simulink model "NDI_and_CA_Model"  (R2012b)
settings: Solver=FixedStepDiscrete  StartTime=0.0  StopTime=inf  FixedStep=T_sim  MaxStep=0.01  RelTol=1e-5
values from neighbouring files (symbols this model uses):
  A_x = 0.015    [SetupComplete.m]
  A_y = A_x    (= 0.015)    [SetupComplete.m]
  A_z = 0.16    [SetupComplete.m]
  C_x = 1.2    [SetupComplete.m]
  C_y = C_x    (= 1.2)    [SetupComplete.m]
  C_z = 2.2    [SetupComplete.m]
  CG_0 = [0,0,0.02]'    [SetupComplete.m]
  eta_23 = deg2rad(-1.42)    [Run3Copter.m]
  g = 9.81    [SetupComplete.m]
  h_M = 0.064    [SetupComplete.m]
  I_BAC_0 = [ Ix,0,Ixz;0,Iy,0;Ixz,0,Iz]    [SetupComplete.m]
  l = 0.345    [SetupComplete.m]
  l_arm = 0.264    [SetupComplete.m]
  m = 3.51    [SetupComplete.m]
  m_0 = 2.61    [SetupComplete.m]
  m_M = 0.300    (= 0.3)    [SetupComplete.m]
  rho = 1.15    [SetupComplete.m]
  Rotation_sign = [ 1,-1,-1]    [SetupComplete.m]
  throtle_1 = 0.512    [Run3Copter.m]
  throtle_23 = throtle_1/cos(eta_23)    [Run3Copter.m]
  Throttle_Hover = X(1)/16    [SetupComplete.m]
libraries: XXCopter_C x24, simulink_extras x21, aerolibutil x3
(part 2 of 2)

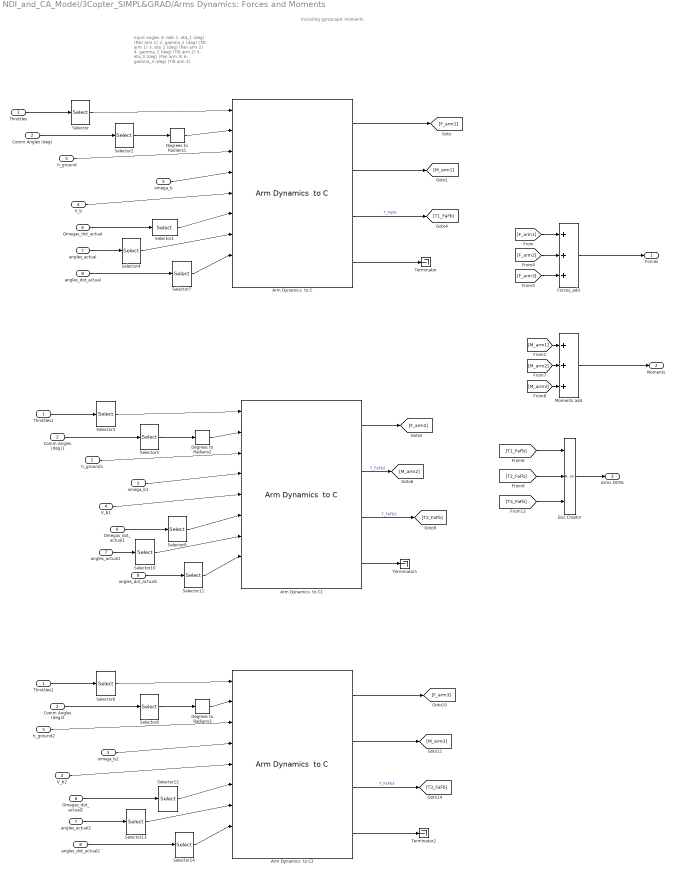
== system NDI_and_CA_Model/3Copter_SIMPL&GRAD/Arms Dynamics: Forces and Moments ==
  note: Including gyroscopic moments
  note: Input angles in rads
      |
      | 1. eta_1 (deg)  (Pan arm 1)
      | 2. gamma_1 (deg)  (Tilt arm 1)
      |
      | 3. eta_2 (deg)  (Pan arm 2)
      | 4. gamma_2 (deg)  (Tilt arm 2)
      |
      | 5. eta_3 (deg)  (Pan arm  3)
      | 6. gamma_3 (deg)  (Tilt arm 3)
  Throttles : Inport
  Comm Angles (deg) : Inport  Port=2
  omega_b : Inport  Port=3
  V_b : Inport  Port=4
  h_ground : Inport  Port=5
  Omegas_dot_actual : Inport  Port=6
  angles_actual : Inport  Port=7
  angles_dot_actual : Inport  Port=8
  Arm Dynamics  to C : XXCopter_C/Arm Dynamics  to C  Rot_sign=Rotation_sign(1)  arm_hub_pos=l*[1;0;0]  Arm_axis=[l_arm;0;0]  arm_num=1  eta_dir=[1;0;0]  gamma_dir=[0;1;0]  J_T=J_T  J_FA=J_FA  h=h  switch_val=direct_feedforward  omega_n=35  xi=1.45  eta_inf_lim=deg2rad(-180)  eta_sup_lim=deg2rad(180)  gamma_inf_lim=deg2rad(-90)  gamma_sup_lim=deg2rad(30)
      link override ESC+Motor Dynamcis  to C/2-D Torque-Throttle-Omega Map: BreakpointsForDimension1=Torque_TTO_vec  BreakpointsForDimension2=Throtle_TTO_vec
  Arm Dynamics  to C1 : XXCopter_C/Arm Dynamics  to C  Rot_sign=Rotation_sign(2)  arm_hub_pos=l*[-1/2;sqrt(3)/2;0]  Arm_axis=[0;l_arm;0]  arm_num=2  eta_dir=[0;1;0]  gamma_dir=[1;0;0]  J_T=J_T  J_FA=J_FA  h=h  switch_val=direct_feedforward  omega_n=35  xi=1.45  eta_inf_lim=deg2rad(-180)  eta_sup_lim=deg2rad(180)  gamma_inf_lim=deg2rad(-30)  gamma_sup_lim=deg2rad(90)
  Arm Dynamics  to C2 : XXCopter_C/Arm Dynamics  to C  Rot_sign=Rotation_sign(3)  arm_hub_pos=l*[-1/2;-sqrt(3)/2;0]  Arm_axis=[0;-l_arm;0]  arm_num=3  eta_dir=[0;1;0]  gamma_dir=[1;0;0]  J_T=J_T  J_FA=J_FA  h=h  switch_val=direct_feedforward  omega_n=35  xi=1.45  eta_inf_lim=deg2rad(-180)  eta_sup_lim=deg2rad(180)  gamma_inf_lim=deg2rad(-90)  gamma_sup_lim=deg2rad(30)
  Bus Creator : BusCreator  Inputs=3
  Comm Angles (deg)1 : InportShadow  Port=2
  Comm Angles (deg)2 : InportShadow  Port=2
  Degrees to Radians1 : simulink_extras/Transformations/Degrees to Radians
  Degrees to Radians2 : simulink_extras/Transformations/Degrees to Radians
  Degrees to Radians3 : simulink_extras/Transformations/Degrees to Radians
  Forces_add : Sum  Inputs=+++
  Moments add : Sum  Inputs=+++
  Omegas_dot_actual1 : InportShadow  Port=6
  Omegas_dot_actual2 : InportShadow  Port=6
  Selector : Selector  IndexMode=Zero-based  InputPortWidth=3  Indices=0
  Selector1 : Selector  IndexMode=Zero-based  InputPortWidth=3  Indices=0
  Selector10 : Selector  IndexMode=Zero-based  InputPortWidth=6  Indices=[2,3]
  Selector11 : Selector  IndexMode=Zero-based  InputPortWidth=6  Indices=[2,3]
  Selector12 : Selector  IndexMode=Zero-based  InputPortWidth=3  Indices=2
  Selector13 : Selector  IndexMode=Zero-based  InputPortWidth=6  Indices=[4,5]
  Selector14 : Selector  IndexMode=Zero-based  InputPortWidth=6  Indices=[4,5]
  Selector2 : Selector  IndexMode=Zero-based  InputPortWidth=6  Indices=[0,1]
  Selector3 : Selector  IndexMode=Zero-based  InputPortWidth=3
  Selector4 : Selector  IndexMode=Zero-based  InputPortWidth=6  Indices=[0,1]
  Selector5 : Selector  IndexMode=Zero-based  InputPortWidth=6  Indices=[2,3]
  Selector6 : Selector  IndexMode=Zero-based  InputPortWidth=3  Indices=2
  Selector7 : Selector  IndexMode=Zero-based  InputPortWidth=6  Indices=[0,1]
  Selector8 : Selector  IndexMode=Zero-based  InputPortWidth=6  Indices=[4,5]
  Selector9 : Selector  IndexMode=Zero-based  InputPortWidth=3
  Terminator : Terminator
  Terminator1 : Terminator
  Terminator2 : Terminator
  Throttles1 : InportShadow
  Throttles2 : InportShadow
  V_b1 : InportShadow  Port=4
  V_b2 : InportShadow  Port=4
  angles_actual1 : InportShadow  Port=7
  angles_actual2 : InportShadow  Port=7
  angles_dot_actual1 : InportShadow  Port=8
  angles_dot_actual2 : InportShadow  Port=8
  h_ground1 : InportShadow  Port=5
  h_ground2 : InportShadow  Port=5
  omega_b1 : InportShadow  Port=3
  omega_b2 : InportShadow  Port=3
  Forces : Outport
  Moments : Outport  Port=2
  Arms DCMs : Outport  Port=3
  wires:
  Throttles/1 -> Selector/1
  Selector/1 -> Arm Dynamics  to C/1
  V_b/1 -> Arm Dynamics  to C/5
  Forces_add/1 -> Forces/1
  Moments add/1 -> Moments/1
  h_ground/1 -> Arm Dynamics  to C/3
  Arm Dynamics  to C/1 -> [F_arm1]
  Arm Dynamics  to C/2 -> [M_arm1]
  [F_arm1] -> Forces_add/1
  [M_arm1] -> Moments add/1
  omega_b/1 -> Arm Dynamics  to C/4
  [F_arm2] -> Forces_add/2
  [F_arm3] -> Forces_add/3
  [M_arm3] -> Moments add/3
  [M_arm2] -> Moments add/2
  Degrees to Radians1/1 -> Arm Dynamics  to C/2
  Comm Angles (deg)/1 -> Selector2/1
  Selector2/1 -> Degrees to Radians1/1
  Arm Dynamics  to C/3 -> [T1_FaFb]  "T_FaFb"
  Throttles1/1 -> Selector3/1
  Selector3/1 -> Arm Dynamics  to C1/1
  V_b1/1 -> Arm Dynamics  to C1/5
  h_ground1/1 -> Arm Dynamics  to C1/3
  omega_b1/1 -> Arm Dynamics  to C1/4
  Degrees to Radians2/1 -> Arm Dynamics  to C1/2
  Comm Angles (deg)1/1 -> Selector5/1
  Selector5/1 -> Degrees to Radians2/1
  Arm Dynamics  to C1/3 -> [T2_FaFb]  "T_FaFb2"
  Throttles2/1 -> Selector6/1
  Selector6/1 -> Arm Dynamics  to C2/1
  V_b2/1 -> Arm Dynamics  to C2/5
  h_ground2/1 -> Arm Dynamics  to C2/3
  Arm Dynamics  to C2/1 -> [F_arm3]
  Arm Dynamics  to C2/2 -> [M_arm3]
  omega_b2/1 -> Arm Dynamics  to C2/4
  Degrees to Radians3/1 -> Arm Dynamics  to C2/2
  Comm Angles (deg)2/1 -> Selector8/1
  Selector8/1 -> Degrees to Radians3/1
  Arm Dynamics  to C2/3 -> [T3_FaFb]  "T_FaFb3"
  Arm Dynamics  to C/4 -> Terminator/1
  Arm Dynamics  to C1/4 -> Terminator1/1
  Arm Dynamics  to C2/4 -> Terminator2/1
  Arm Dynamics  to C1/1 -> [F_arm2]
  Arm Dynamics  to C1/2 -> [M_arm2]  "T_FaFb2"
  Bus Creator/1 -> Arms DCMs/1
  [T1_FaFb] -> Bus Creator/1
  [T2_FaFb] -> Bus Creator/2
  [T3_FaFb] -> Bus Creator/3
  Omegas_dot_actual/1 -> Selector1/1
  Selector1/1 -> Arm Dynamics  to C/6
  angles_actual/1 -> Selector4/1
  Selector4/1 -> Arm Dynamics  to C/7
  angles_dot_actual/1 -> Selector7/1
  Selector7/1 -> Arm Dynamics  to C/8
  Omegas_dot_actual1/1 -> Selector9/1
  Selector9/1 -> Arm Dynamics  to C1/6
  Selector10/1 -> Arm Dynamics  to C1/7
  angles_dot_actual1/1 -> Selector11/1
  angles_actual1/1 -> Selector10/1
  Selector11/1 -> Arm Dynamics  to C1/8
  Omegas_dot_actual2/1 -> Selector12/1
  Selector12/1 -> Arm Dynamics  to C2/6
  Selector13/1 -> Arm Dynamics  to C2/7
  angles_dot_actual2/1 -> Selector14/1
  angles_actual2/1 -> Selector13/1
  Selector14/1 -> Arm Dynamics  to C2/8

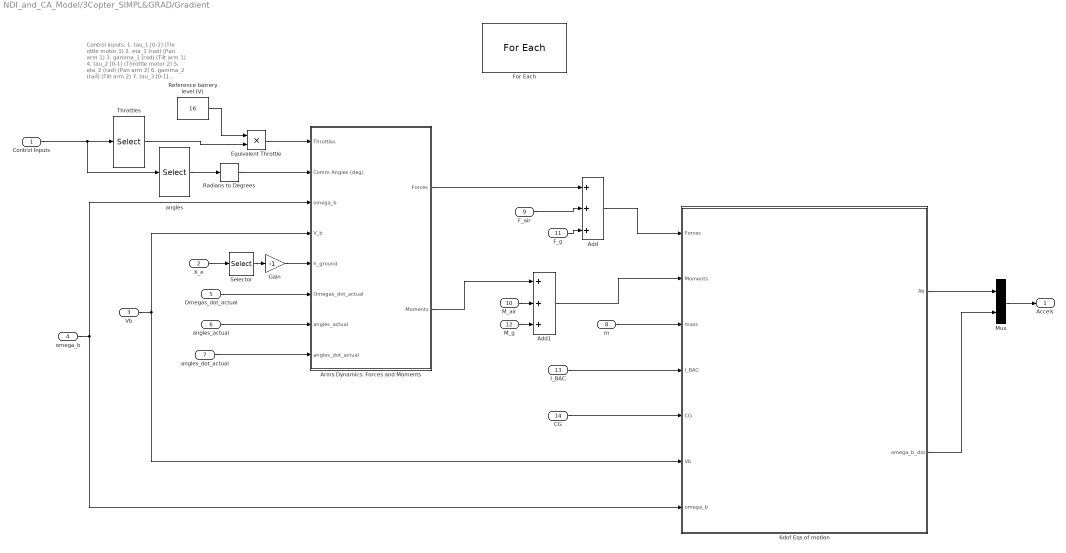
== system NDI_and_CA_Model/3Copter_SIMPL&GRAD/Gradient ==
  note: Control inputs:
      | 1. tau_1 [0-1] (Thr ottle motor 1)
      | 2. eta_1 (rad)  (Pan arm 1)
      | 3. gamma_1 (rad)  (Tilt arm 1)
      |
      | 4. tau_2 [0-1] (Throttle motor 2)
      | 5. eta_2 (rad)  (Pan arm 2)
      | 6. gamma_2 (rad)  (Tilt arm 2)
      |
      | 7. tau_3 [0-1] (Throttle motor 3)
      | 8. eta_3 (rad)  (Pan arm  3)
      | 9. gamma_3 (rad)  (Tilt arm 3)
  "Control Inputs " : Inport  Partition=on  PartitionDimension=1  PartitionWidth=9
  X_e : Inport  Port=2  Partition=off
  Vb : Inport  Port=3  Partition=off
  omega_b : Inport  Port=4  Partition=off
  Omegas_dot_actual : Inport  Port=5  Partition=off
  angles_actual : Inport  Port=6  Partition=off
  angles_dot_actual : Inport  Port=7  Partition=off
  " m" : Inport  Port=8  Partition=off
  F_air : Inport  Port=9  Partition=off
  M_air : Inport  Port=10  Partition=off
  F_g : Inport  Port=11  Partition=off
  M_g : Inport  Port=12  Partition=off
  I_BAC : Inport  Port=13  Partition=off
  CG : Inport  Port=14  Partition=off
  6dof Eqs of motion : Subsystem  TreatAsAtomicUnit=on
  Add : Sum  Inputs=+++
  Add1 : Sum  Inputs=+++
  Arms Dynamics: Forces and Moments : Subsystem  TreatAsAtomicUnit=on
  Equivalent Throttle : Product  Inputs=**
  For Each : ForEach  DisableCoverage=on  IndexMode=One-based
  Gain : Gain  Gain=-1
  Mux : Mux  Inputs=[3,3]
  Radians to Degrees : simulink_extras/Transformations/Radians to Degrees
  Reference batrery level (V) : Constant  Value=16
  Selector : Selector  IndexMode=Zero-based  InputPortWidth=3  Indices=2
  Throttles : Selector  IndexMode=Zero-based  InputPortWidth=9  Indices=[0,3,6]
  "angles " : Selector  IndexMode=Zero-based  InputPortWidth=9  Indices=[1,2,4,5,7,8]
  Accels : Outport  ConcatenationDimension=2
  wires:
  " m"/1 -> 6dof Eqs of motion/3(mass)
  Vb/1 -> 6dof Eqs of motion/6(Vb), Arms Dynamics: Forces and Moments/4(V_b)
  omega_b/1 -> Arms Dynamics: Forces and Moments/3(omega_b), 6dof Eqs of motion/7(omega_b)
  X_e/1 -> Selector/1
  Selector/1 -> Gain/1
  Gain/1 -> Arms Dynamics: Forces and Moments/5(h_ground)
  F_air/1 -> Add/2
  Arms Dynamics: Forces and Moments/1(Forces) -> Add/1
  F_g/1 -> Add/3
  Arms Dynamics: Forces and Moments/2(Moments) -> Add1/1
  M_g/1 -> Add1/3
  M_air/1 -> Add1/2
  Throttles/1 -> Equivalent Throttle/2
  "Control Inputs "/1 -> Throttles/1, "angles "/1
  "angles "/1 -> Radians to Degrees/1
  Add/1 -> 6dof Eqs of motion/1(Forces)
  CG/1 -> 6dof Eqs of motion/5(CG)
  I_BAC/1 -> 6dof Eqs of motion/4(I_BAC)
  Equivalent Throttle/1 -> Arms Dynamics: Forces and Moments/1(Throttles)
  Reference batrery level (V)/1 -> Equivalent Throttle/1
  Add1/1 -> 6dof Eqs of motion/2(Moments)
  6dof Eqs of motion/2(omega_b_dot) -> Mux/2
  Omegas_dot_actual/1 -> Arms Dynamics: Forces and Moments/6(Omegas_dot_actual)
  angles_dot_actual/1 -> Arms Dynamics: Forces and Moments/8(angles_dot_actual)
  angles_actual/1 -> Arms Dynamics: Forces and Moments/7(angles_actual)
  6dof Eqs of motion/1(Ab) -> Mux/1
  Mux/1 -> Accels/1
  Radians to Degrees/1 -> Arms Dynamics: Forces and Moments/2(Comm Angles (deg))

== system NDI_and_CA_Model/3Copter_SIMPL&GRAD/Mass Properties ==
  Arms DCMs : Inport
  CG_0 : Inport  Port=2
  m_0 : Inport  Port=3
  m : Inport  Port=4
  m_M : Inport  Port=5
  I_BAC_0 : Inport  Port=6
  Arm Inertia : MATLAB Function  TreatAsAtomicUnit=on
      settings: PermitHierarchicalResolution=ParametersOnly
  Bus Selector : BusSelector  OutputSignals=T_FaFb,T_FaFb2,T_FaFb3
  CG position : Sum
  Divide : Product  Inputs=*/
  Divide1 : Product  Inputs=**
  Divide2 : Product  Inputs=/*
  Divide3 : Product  Inputs=**
  Motors Pos sum : Sum  Inputs=+++
  Total I_BAC : Sum
  I_BAC : Outport
  CG : Outport  Port=2
  wires:
  Arms DCMs/1 -> Bus Selector/1
  Bus Selector/3 -> Arm Inertia/3(T3_FAFb)  "<T_FaFb3>"
  Bus Selector/2 -> Arm Inertia/2(T2_FAFb)  "<T_FaFb2>"
  Bus Selector/1 -> Arm Inertia/1(T1_FAFb)  "<T_FaFb>"
  Total I_BAC/1 -> I_BAC/1
  m_0/1 -> Divide/1
  m/1 -> Divide/2, Divide2/1
  CG_0/1 -> Divide1/1
  Divide/1 -> Divide1/2
  m_M/1 -> Divide2/2
  CG position/1 -> CG/1
  Divide1/1 -> CG position/1
  Motors Pos sum/1 -> Divide3/1
  Divide2/1 -> Divide3/2
  Divide3/1 -> CG position/2
  Arm Inertia/3(r2_M) -> Motors Pos sum/2
  Arm Inertia/4(r3_M) -> Motors Pos sum/1
  Arm Inertia/1(I_M) -> Total I_BAC/2
  I_BAC_0/1 -> Total I_BAC/1
  Arm Inertia/2(r1_M) -> Motors Pos sum/3

== system NDI_and_CA_Model/3Copter_SIMPL&GRAD/Normalize Quaternion ==
  q : Inport
  Demux : Demux
  Math Function : Math  Operator=reciprocal  SaturateOnIntegerOverflow=on
  Mux : Mux
  Product{,1..3} (4 alike) : Product  Inputs=**
  Quaternion Modulus : aerolibutil/Quaternion Modulus
  normal(q) : Outport
  wires:
  Product3/1 -> Mux/4
  Product2/1 -> Mux/3
  Product1/1 -> Mux/2
  Product/1 -> Mux/1
  Quaternion Modulus/1 -> Math Function/1
  q/1 -> Demux/1, Quaternion Modulus/1
  Mux/1 -> normal(q)/1
  Demux/1 -> Product/1
  Demux/2 -> Product1/1
  Demux/3 -> Product2/1
  Demux/4 -> Product3/1
  Math Function/1 -> Product3/2, Product2/2, Product/2, Product1/2

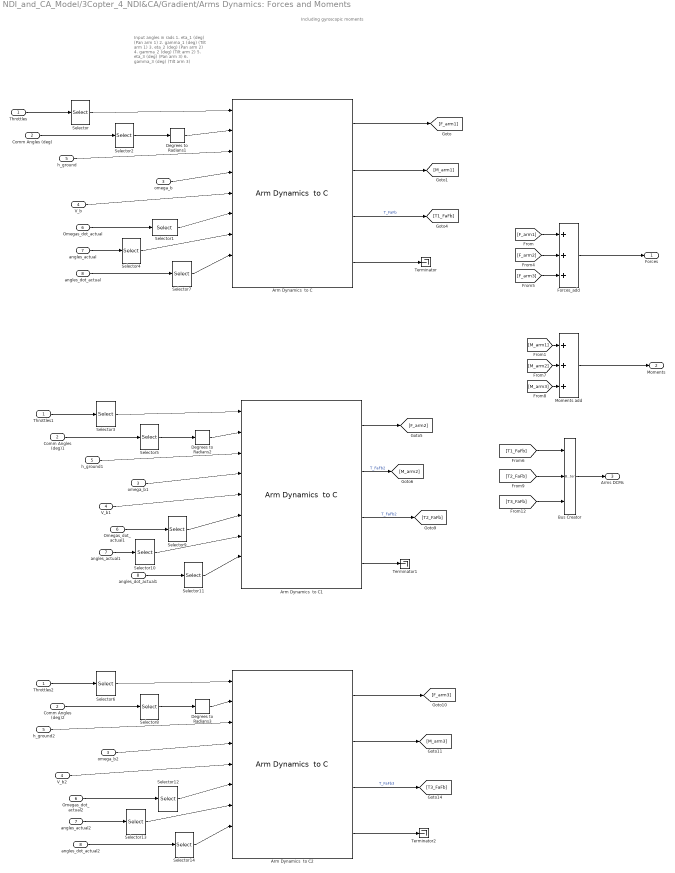
== system NDI_and_CA_Model/3Copter_4_NDI&CA/Gradient/Arms Dynamics: Forces and Moments ==
  note: Including gyroscopic moments
  note: Input angles in rads
      |
      | 1. eta_1 (deg)  (Pan arm 1)
      | 2. gamma_1 (deg)  (Tilt arm 1)
      |
      | 3. eta_2 (deg)  (Pan arm 2)
      | 4. gamma_2 (deg)  (Tilt arm 2)
      |
      | 5. eta_3 (deg)  (Pan arm  3)
      | 6. gamma_3 (deg)  (Tilt arm 3)
  Throttles : Inport
  Comm Angles (deg) : Inport  Port=2
  omega_b : Inport  Port=3
  V_b : Inport  Port=4
  h_ground : Inport  Port=5
  Omegas_dot_actual : Inport  Port=6
  angles_actual : Inport  Port=7
  angles_dot_actual : Inport  Port=8
  Arm Dynamics  to C : XXCopter_C/Arm Dynamics  to C  Rot_sign=Rotation_sign(1)  arm_hub_pos=l*[1;0;0]  Arm_axis=[l_arm;0;0]  arm_num=1  eta_dir=[1;0;0]  gamma_dir=[0;1;0]  J_T=J_T  J_FA=J_FA  h=h  switch_val=direct_feedforward  omega_n=35  xi=1.45  eta_inf_lim=deg2rad(-180)  eta_sup_lim=deg2rad(180)  gamma_inf_lim=deg2rad(-90)  gamma_sup_lim=deg2rad(30)
      link override ESC+Motor Dynamcis  to C/2-D Torque-Throttle-Omega Map: BreakpointsForDimension1=Torque_TTO_vec  BreakpointsForDimension2=Throtle_TTO_vec
  Arm Dynamics  to C1 : XXCopter_C/Arm Dynamics  to C  Rot_sign=Rotation_sign(2)  arm_hub_pos=l*[-1/2;sqrt(3)/2;0]  Arm_axis=[0;l_arm;0]  arm_num=2  eta_dir=[0;1;0]  gamma_dir=[1;0;0]  J_T=J_T  J_FA=J_FA  h=h  switch_val=direct_feedforward  omega_n=35  xi=1.45  eta_inf_lim=deg2rad(-180)  eta_sup_lim=deg2rad(180)  gamma_inf_lim=deg2rad(-30)  gamma_sup_lim=deg2rad(90)
  Arm Dynamics  to C2 : XXCopter_C/Arm Dynamics  to C  Rot_sign=Rotation_sign(3)  arm_hub_pos=l*[-1/2;-sqrt(3)/2;0]  Arm_axis=[0;-l_arm;0]  arm_num=3  eta_dir=[0;1;0]  gamma_dir=[1;0;0]  J_T=J_T  J_FA=J_FA  h=h  switch_val=direct_feedforward  omega_n=35  xi=1.45  eta_inf_lim=deg2rad(-180)  eta_sup_lim=deg2rad(180)  gamma_inf_lim=deg2rad(-90)  gamma_sup_lim=deg2rad(30)
  Bus Creator : BusCreator  Inputs=3
  Comm Angles (deg)1 : InportShadow  Port=2
  Comm Angles (deg)2 : InportShadow  Port=2
  Degrees to Radians1 : simulink_extras/Transformations/Degrees to Radians
  Degrees to Radians2 : simulink_extras/Transformations/Degrees to Radians
  Degrees to Radians3 : simulink_extras/Transformations/Degrees to Radians
  Forces_add : Sum  Inputs=+++
  Moments add : Sum  Inputs=+++
  Omegas_dot_actual1 : InportShadow  Port=6
  Omegas_dot_actual2 : InportShadow  Port=6
  Selector : Selector  IndexMode=Zero-based  InputPortWidth=3  Indices=0
  Selector1 : Selector  IndexMode=Zero-based  InputPortWidth=3  Indices=0
  Selector10 : Selector  IndexMode=Zero-based  InputPortWidth=6  Indices=[2,3]
  Selector11 : Selector  IndexMode=Zero-based  InputPortWidth=6  Indices=[2,3]
  Selector12 : Selector  IndexMode=Zero-based  InputPortWidth=3  Indices=2
  Selector13 : Selector  IndexMode=Zero-based  InputPortWidth=6  Indices=[4,5]
  Selector14 : Selector  IndexMode=Zero-based  InputPortWidth=6  Indices=[4,5]
  Selector2 : Selector  IndexMode=Zero-based  InputPortWidth=6  Indices=[0,1]
  Selector3 : Selector  IndexMode=Zero-based  InputPortWidth=3
  Selector4 : Selector  IndexMode=Zero-based  InputPortWidth=6  Indices=[0,1]
  Selector5 : Selector  IndexMode=Zero-based  InputPortWidth=6  Indices=[2,3]
  Selector6 : Selector  IndexMode=Zero-based  InputPortWidth=3  Indices=2
  Selector7 : Selector  IndexMode=Zero-based  InputPortWidth=6  Indices=[0,1]
  Selector8 : Selector  IndexMode=Zero-based  InputPortWidth=6  Indices=[4,5]
  Selector9 : Selector  IndexMode=Zero-based  InputPortWidth=3
  Terminator : Terminator
  Terminator1 : Terminator
  Terminator2 : Terminator
  Throttles1 : InportShadow
  Throttles2 : InportShadow
  V_b1 : InportShadow  Port=4
  V_b2 : InportShadow  Port=4
  angles_actual1 : InportShadow  Port=7
  angles_actual2 : InportShadow  Port=7
  angles_dot_actual1 : InportShadow  Port=8
  angles_dot_actual2 : InportShadow  Port=8
  h_ground1 : InportShadow  Port=5
  h_ground2 : InportShadow  Port=5
  omega_b1 : InportShadow  Port=3
  omega_b2 : InportShadow  Port=3
  Forces : Outport
  Moments : Outport  Port=2
  Arms DCMs : Outport  Port=3
  wires:
  Throttles/1 -> Selector/1
  Selector/1 -> Arm Dynamics  to C/1
  V_b/1 -> Arm Dynamics  to C/5
  Forces_add/1 -> Forces/1
  Moments add/1 -> Moments/1
  h_ground/1 -> Arm Dynamics  to C/3
  Arm Dynamics  to C/1 -> [F_arm1]
  Arm Dynamics  to C/2 -> [M_arm1]
  [F_arm1] -> Forces_add/1
  [M_arm1] -> Moments add/1
  omega_b/1 -> Arm Dynamics  to C/4
  [F_arm2] -> Forces_add/2
  [F_arm3] -> Forces_add/3
  [M_arm3] -> Moments add/3
  [M_arm2] -> Moments add/2
  Degrees to Radians1/1 -> Arm Dynamics  to C/2
  Comm Angles (deg)/1 -> Selector2/1
  Selector2/1 -> Degrees to Radians1/1
  Arm Dynamics  to C/3 -> [T1_FaFb]  "T_FaFb"
  Throttles1/1 -> Selector3/1
  Selector3/1 -> Arm Dynamics  to C1/1
  V_b1/1 -> Arm Dynamics  to C1/5
  h_ground1/1 -> Arm Dynamics  to C1/3
  omega_b1/1 -> Arm Dynamics  to C1/4
  Degrees to Radians2/1 -> Arm Dynamics  to C1/2
  Comm Angles (deg)1/1 -> Selector5/1
  Selector5/1 -> Degrees to Radians2/1
  Arm Dynamics  to C1/3 -> [T2_FaFb]  "T_FaFb2"
  Throttles2/1 -> Selector6/1
  Selector6/1 -> Arm Dynamics  to C2/1
  V_b2/1 -> Arm Dynamics  to C2/5
  h_ground2/1 -> Arm Dynamics  to C2/3
  Arm Dynamics  to C2/1 -> [F_arm3]
  Arm Dynamics  to C2/2 -> [M_arm3]
  omega_b2/1 -> Arm Dynamics  to C2/4
  Degrees to Radians3/1 -> Arm Dynamics  to C2/2
  Comm Angles (deg)2/1 -> Selector8/1
  Selector8/1 -> Degrees to Radians3/1
  Arm Dynamics  to C2/3 -> [T3_FaFb]  "T_FaFb3"
  Arm Dynamics  to C/4 -> Terminator/1
  Arm Dynamics  to C1/4 -> Terminator1/1
  Arm Dynamics  to C2/4 -> Terminator2/1
  Arm Dynamics  to C1/1 -> [F_arm2]
  Arm Dynamics  to C1/2 -> [M_arm2]  "T_FaFb2"
  Bus Creator/1 -> Arms DCMs/1
  [T1_FaFb] -> Bus Creator/1
  [T2_FaFb] -> Bus Creator/2
  [T3_FaFb] -> Bus Creator/3
  Omegas_dot_actual/1 -> Selector1/1
  Selector1/1 -> Arm Dynamics  to C/6
  angles_actual/1 -> Selector4/1
  Selector4/1 -> Arm Dynamics  to C/7
  angles_dot_actual/1 -> Selector7/1
  Selector7/1 -> Arm Dynamics  to C/8
  Omegas_dot_actual1/1 -> Selector9/1
  Selector9/1 -> Arm Dynamics  to C1/6
  Selector10/1 -> Arm Dynamics  to C1/7
  angles_dot_actual1/1 -> Selector11/1
  angles_actual1/1 -> Selector10/1
  Selector11/1 -> Arm Dynamics  to C1/8
  Omegas_dot_actual2/1 -> Selector12/1
  Selector12/1 -> Arm Dynamics  to C2/6
  Selector13/1 -> Arm Dynamics  to C2/7
  angles_dot_actual2/1 -> Selector14/1
  angles_actual2/1 -> Selector13/1
  Selector14/1 -> Arm Dynamics  to C2/8

== system NDI_and_CA_Model/3Copter_4_SIMPL/6dof Eqs of motion/q_dot ==
  omega_b : Inport
  q : Inport  Port=2
  Quaternion_dot : MATLAB Function  TreatAsAtomicUnit=on  VariantObject=Variant
      settings: PermitHierarchicalResolution=ParametersOnly
  q_dot : Outport
  wires:
  omega_b/1 -> Quaternion_dot/1(omega_b)  "omega_b"
  q/1 -> Quaternion_dot/2(q)  "q"
  Quaternion_dot/1(q_dot) -> q_dot/1

== system NDI_and_CA_Model/3Copter_SIMPL&GRAD/Gradient/6dof Eqs of motion ==
  Forces : Inport
  Moments : Inport  Port=2
  mass : Inport  Port=3
  I_BAC : Inport  Port=4
  CG : Inport  Port=5
  Vb : Inport  Port=6
  omega_b : Inport  Port=7
  Rotational Eq : XXCopter_C/Rotational Eq
  Translational_Eq : XXCopter_C/Translational_Eq
  Ab : Outport  PortDimensions=[3,1]
  omega_b_dot : Outport  Port=2
  wires:
  I_BAC/1 -> Rotational Eq/3
  mass/1 -> Translational_Eq/5
  Forces/1 -> Translational_Eq/4
  omega_b/1 -> Translational_Eq/2, Rotational Eq/1
  Rotational Eq/1 -> Translational_Eq/3, omega_b_dot/1
  Translational_Eq/1 -> Ab/1  "A_b"
  CG/1 -> Translational_Eq/6
  Moments/1 -> Rotational Eq/2
  Vb/1 -> Translational_Eq/1

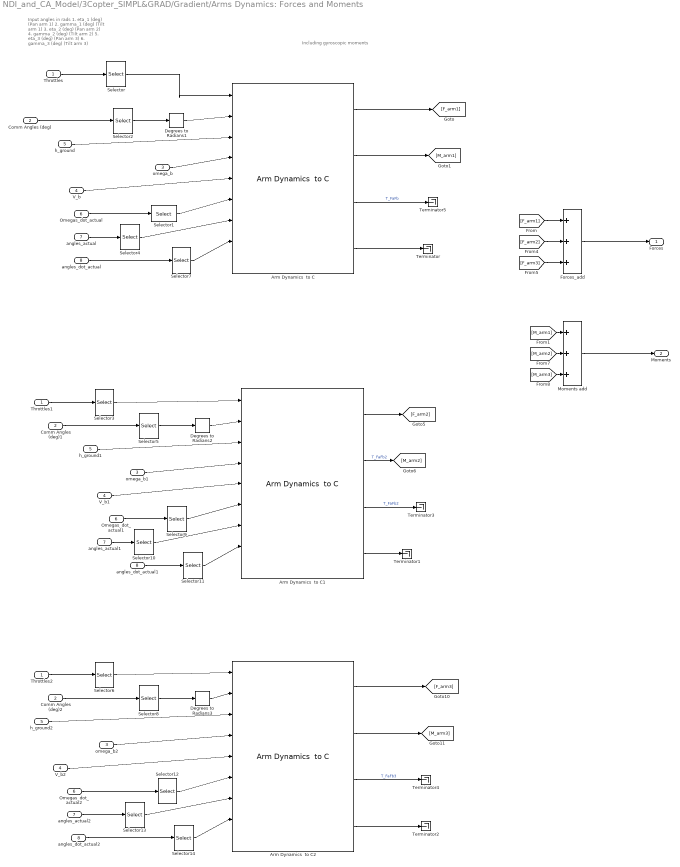
== system NDI_and_CA_Model/3Copter_SIMPL&GRAD/Gradient/Arms Dynamics: Forces and Moments ==
  note: Including gyroscopic moments
  note: Input angles in rads
      |
      | 1. eta_1 (deg)  (Pan arm 1)
      | 2. gamma_1 (deg)  (Tilt arm 1)
      |
      | 3. eta_2 (deg)  (Pan arm 2)
      | 4. gamma_2 (deg)  (Tilt arm 2)
      |
      | 5. eta_3 (deg)  (Pan arm  3)
      | 6. gamma_3 (deg)  (Tilt arm 3)
  Throttles : Inport
  Comm Angles (deg) : Inport  Port=2
  omega_b : Inport  Port=3
  V_b : Inport  Port=4
  h_ground : Inport  Port=5
  Omegas_dot_actual : Inport  Port=6
  angles_actual : Inport  Port=7
  angles_dot_actual : Inport  Port=8
  Arm Dynamics  to C : XXCopter_C/Arm Dynamics  to C  Rot_sign=Rotation_sign(1)  arm_hub_pos=l*[1;0;0]  Arm_axis=[l_arm;0;0]  arm_num=1  eta_dir=[1;0;0]  gamma_dir=[0;1;0]  J_T=J_T  J_FA=J_FA  h=h  switch_val=direct_feedforward  omega_n=35  xi=1.45  eta_inf_lim=deg2rad(-180)  eta_sup_lim=deg2rad(180)  gamma_inf_lim=deg2rad(-90)  gamma_sup_lim=deg2rad(30)
      link override ESC+Motor Dynamcis  to C/2-D Torque-Throttle-Omega Map: BreakpointsForDimension1=Torque_TTO_vec  BreakpointsForDimension2=Throtle_TTO_vec
  Arm Dynamics  to C1 : XXCopter_C/Arm Dynamics  to C  Rot_sign=Rotation_sign(2)  arm_hub_pos=l*[-1/2;sqrt(3)/2;0]  Arm_axis=[l_arm;0;0]  arm_num=2  eta_dir=[0;1;0]  gamma_dir=[1;0;0]  J_T=J_T  J_FA=J_FA  h=h  switch_val=direct_feedforward  omega_n=35  xi=1.45  eta_inf_lim=deg2rad(-180)  eta_sup_lim=deg2rad(180)  gamma_inf_lim=deg2rad(-30)  gamma_sup_lim=deg2rad(90)
  Arm Dynamics  to C2 : XXCopter_C/Arm Dynamics  to C  Rot_sign=Rotation_sign(3)  arm_hub_pos=l*[-1/2;-sqrt(3)/2;0]  Arm_axis=[l_arm;0;0]  arm_num=3  eta_dir=[0;1;0]  gamma_dir=[1;0;0]  J_T=J_T  J_FA=J_FA  h=h  switch_val=direct_feedforward  omega_n=35  xi=1.45  eta_inf_lim=deg2rad(-180)  eta_sup_lim=deg2rad(180)  gamma_inf_lim=deg2rad(-90)  gamma_sup_lim=deg2rad(30)
  Comm Angles (deg)1 : InportShadow  Port=2
  Comm Angles (deg)2 : InportShadow  Port=2
  Degrees to Radians1 : simulink_extras/Transformations/Degrees to Radians
  Degrees to Radians2 : simulink_extras/Transformations/Degrees to Radians
  Degrees to Radians3 : simulink_extras/Transformations/Degrees to Radians
  Forces_add : Sum  Inputs=+++
  Moments add : Sum  Inputs=+++
  Omegas_dot_actual1 : InportShadow  Port=6
  Omegas_dot_actual2 : InportShadow  Port=6
  Selector : Selector  IndexMode=Zero-based  InputPortWidth=3  Indices=0
  Selector1 : Selector  IndexMode=Zero-based  InputPortWidth=3  Indices=0
  Selector10 : Selector  IndexMode=Zero-based  InputPortWidth=6  Indices=[2,3]
  Selector11 : Selector  IndexMode=Zero-based  InputPortWidth=6  Indices=[2,3]
  Selector12 : Selector  IndexMode=Zero-based  InputPortWidth=3  Indices=2
  Selector13 : Selector  IndexMode=Zero-based  InputPortWidth=6  Indices=[4,5]
  Selector14 : Selector  IndexMode=Zero-based  InputPortWidth=6  Indices=[4,5]
  Selector2 : Selector  IndexMode=Zero-based  InputPortWidth=6  Indices=[0,1]
  Selector3 : Selector  IndexMode=Zero-based  InputPortWidth=3
  Selector4 : Selector  IndexMode=Zero-based  InputPortWidth=6  Indices=[0,1]
  Selector5 : Selector  IndexMode=Zero-based  InputPortWidth=6  Indices=[2,3]
  Selector6 : Selector  IndexMode=Zero-based  InputPortWidth=3  Indices=2
  Selector7 : Selector  IndexMode=Zero-based  InputPortWidth=6  Indices=[0,1]
  Selector8 : Selector  IndexMode=Zero-based  InputPortWidth=6  Indices=[4,5]
  Selector9 : Selector  IndexMode=Zero-based  InputPortWidth=3
  Terminator{,1..5} (6 alike) : Terminator
  Throttles1 : InportShadow
  Throttles2 : InportShadow
  V_b1 : InportShadow  Port=4
  V_b2 : InportShadow  Port=4
  angles_actual1 : InportShadow  Port=7
  angles_actual2 : InportShadow  Port=7
  angles_dot_actual1 : InportShadow  Port=8
  angles_dot_actual2 : InportShadow  Port=8
  h_ground1 : InportShadow  Port=5
  h_ground2 : InportShadow  Port=5
  omega_b1 : InportShadow  Port=3
  omega_b2 : InportShadow  Port=3
  Forces : Outport
  Moments : Outport  Port=2
  wires:
  Throttles/1 -> Selector/1
  Selector/1 -> Arm Dynamics  to C/1
  V_b/1 -> Arm Dynamics  to C/5
  Forces_add/1 -> Forces/1
  Moments add/1 -> Moments/1
  h_ground/1 -> Arm Dynamics  to C/3
  Arm Dynamics  to C/1 -> [F_arm1]
  Arm Dynamics  to C/2 -> [M_arm1]
  [F_arm1] -> Forces_add/1
  [M_arm1] -> Moments add/1
  omega_b/1 -> Arm Dynamics  to C/4
  [F_arm2] -> Forces_add/2
  [F_arm3] -> Forces_add/3
  [M_arm3] -> Moments add/3
  [M_arm2] -> Moments add/2
  Degrees to Radians1/1 -> Arm Dynamics  to C/2
  Comm Angles (deg)/1 -> Selector2/1
  Selector2/1 -> Degrees to Radians1/1
  Arm Dynamics  to C/3 -> Terminator5/1  "T_FaFb"
  Throttles1/1 -> Selector3/1
  Selector3/1 -> Arm Dynamics  to C1/1
  V_b1/1 -> Arm Dynamics  to C1/5
  h_ground1/1 -> Arm Dynamics  to C1/3
  omega_b1/1 -> Arm Dynamics  to C1/4
  Degrees to Radians2/1 -> Arm Dynamics  to C1/2
  Comm Angles (deg)1/1 -> Selector5/1
  Selector5/1 -> Degrees to Radians2/1
  Arm Dynamics  to C1/3 -> Terminator3/1  "T_FaFb2"
  Throttles2/1 -> Selector6/1
  Selector6/1 -> Arm Dynamics  to C2/1
  V_b2/1 -> Arm Dynamics  to C2/5
  h_ground2/1 -> Arm Dynamics  to C2/3
  Arm Dynamics  to C2/1 -> [F_arm3]
  Arm Dynamics  to C2/2 -> [M_arm3]
  omega_b2/1 -> Arm Dynamics  to C2/4
  Degrees to Radians3/1 -> Arm Dynamics  to C2/2
  Comm Angles (deg)2/1 -> Selector8/1
  Selector8/1 -> Degrees to Radians3/1
  Arm Dynamics  to C2/3 -> Terminator4/1  "T_FaFb3"
  Arm Dynamics  to C/4 -> Terminator/1
  Arm Dynamics  to C1/4 -> Terminator1/1
  Arm Dynamics  to C2/4 -> Terminator2/1
  Arm Dynamics  to C1/1 -> [F_arm2]
  Arm Dynamics  to C1/2 -> [M_arm2]  "T_FaFb2"
  Omegas_dot_actual/1 -> Selector1/1
  Selector1/1 -> Arm Dynamics  to C/6
  angles_actual/1 -> Selector4/1
  Selector4/1 -> Arm Dynamics  to C/7
  angles_dot_actual/1 -> Selector7/1
  Selector7/1 -> Arm Dynamics  to C/8
  Omegas_dot_actual1/1 -> Selector9/1
  Selector9/1 -> Arm Dynamics  to C1/6
  Selector10/1 -> Arm Dynamics  to C1/7
  angles_dot_actual1/1 -> Selector11/1
  angles_actual1/1 -> Selector10/1
  Selector11/1 -> Arm Dynamics  to C1/8
  Omegas_dot_actual2/1 -> Selector12/1
  Selector12/1 -> Arm Dynamics  to C2/6
  Selector13/1 -> Arm Dynamics  to C2/7
  angles_dot_actual2/1 -> Selector14/1
  angles_actual2/1 -> Selector13/1
  Selector14/1 -> Arm Dynamics  to C2/8

== matlab function NDI_and_CA_Model/3Copter_SIMPL&GRAD/Get gradient ==
  data: epsilon input; CA_Grad output; Perturb_evaluations input
function CA_Grad  = Get_gradient(epsilon,Perturb_evaluations)

CA_Grad = zeros(6,9);

for i=1:9
    CA_Grad(:,i)= ( Perturb_evaluations(:,2*i)-Perturb_evaluations(:,2*i-1)  )./(epsilon);
end






end

== matlab function NDI_and_CA_Model/3Copter_SIMPL&GRAD/Perturbations ==
  data: Ctrl_input_rad output; epsilon input; Ctrl_input_deg input; Pert_Ctrl_rad output
function [Ctrl_input_rad,Pert_Ctrl_rad] = Perturbate_input(epsilon, Ctrl_input_deg)
% The control input has a dimension of 9
% The gradient is computed with 2 evaluations, so the output vector has
% 2*9*9 variables

Ctrl_input_rad = Ctrl_input_deg;
Ctrl_input_rad(2:3,1) = deg2rad( Ctrl_input_deg(2:3,1) );
Ctrl_input_rad(5:6,1) = deg2rad( Ctrl_input_deg(5:6,1) );
Ctrl_input_rad(8:9,1) = deg2rad( Ctrl_input_deg(8:9,1) );

Pert_Ctrl_rad=zeros(2*9*9,1);

for i=1:9
    % Left
    tmp=Ctrl_input_rad;
    tmp(i)=tmp(i)-epsilon;
    Pert_Ctrl_rad( 1+2*(i-1)*9:(2*i-1)*9 ) = tmp;
    % Right
    tmp=Ctrl_input_rad;
    tmp(i)=tmp(i)+epsilon;
    Pert_Ctrl_rad( 1+(2*i-1)*9 :2*i*9 ) = tmp;
end






end

== matlab function NDI_and_CA_Model/3Copter_4_SIMPL/6dof Eqs of motion/q_dot/Quaternion_dot ==
  data: omega_b input; q_dot output; q input
function q_dot = Quaternion_dot(omega_b,q)


q_dot = 1/2*HamiltonProduct(q,[0;omega_b]);

== matlab function NDI_and_CA_Model/3Copter_4_NDI&CA/Aerodynamics body Force and Moment1 ==
  data: V_b input; F_a_b output; M_a_b output; rho parameter; C_x parameter; C_y parameter; C_z parameter; A_x parameter; A_y parameter; A_z parameter
function [F_a_b,M_a_b]   = Aero_body_Forces_and_Mom( V_b, rho,C_x,C_y,C_z,A_x,A_y,A_z)


F_a_b=1/2.0*rho*(V_b*V_b')*[C_x*A_x;C_y*A_y;C_z*A_z].*( - V_b./(norm(V_b)+eps) );
M_a_b=[0;0;0];
end

== matlab function NDI_and_CA_Model/3Copter_4_SIMPL/Aerodynamics body Force and Moment1 ==
  data: V_b input; F_a_b output; M_a_b output; rho parameter; C_x parameter; C_y parameter; C_z parameter; A_x parameter; A_y parameter; A_z parameter
function [F_a_b,M_a_b]   = Aero_body_Forces_and_Mom( V_b, rho,C_x,C_y,C_z,A_x,A_y,A_z)


F_a_b=1/2.0*rho*(V_b*V_b')*[C_x*A_x;C_y*A_y;C_z*A_z].*( - V_b./(norm(V_b)+eps) );
M_a_b=[0;0;0];
end

== matlab function NDI_and_CA_Model/3Copter_4_NDI&CA/Get gradient ==
  data: epsilon input; CA_Grad output; Perturb_evaluations input
function CA_Grad  = Get_gradient(epsilon,Perturb_evaluations)

CA_Grad = zeros(6,9);

for i=1:9
    CA_Grad(:,i)= ( Perturb_evaluations(:,2*i)-Perturb_evaluations(:,2*i-1)  )./(epsilon);
end






end

== matlab function NDI_and_CA_Model/3Copter_4_NDI&CA/Mass Properties/Arm Inertia ==
  data: T1_FAFb input; T2_FAFb input; T3_FAFb input; I_M output; l parameter; h_M parameter; m_M parameter; r1_M output; r2_M output; r3_M output
function [I_M,r1_M,r2_M,r3_M]  = Arm1_inertia(T1_FAFb,T2_FAFb,T3_FAFb, l, h_M, m_M)


r1_M=[l;0;0]+T1_FAFb*[0;0;-h_M];
r2_M=[-1/2*l;sqrt(3)/2*l;0]+T2_FAFb*[0;0;-h_M];
r3_M=[-1/2*l;-sqrt(3)/2*l;0]+T3_FAFb*[0;0;-h_M];


I_M1 = m_M*[ r1_M(2)^2+r1_M(3)^2,r1_M(1)*r1_M(2),r1_M(1)*r1_M(3);...
            r1_M(1)*r1_M(2), r1_M(1)^2+r1_M(3)^2, r1_M(2)*r1_M(3);...
            r1_M(1)*r1_M(3),r1_M(2)*r1_M(3), r1_M(1)^2+r1_M(2)^2];
I_M2 = m_M*[ r2_M(2)^2+r2_M(3)^2,r2_M(1)*r2_M(2),r2_M(1)*r2_M(3);...
            r2_M(1)*r2_M(2), r2_M(1)^2+r2_M(3)^2, r2_M(2)*r2_M(3);...
            r2_M(1)*r2_M(3),r2_M(2)*r2_M(3), r2_M(1)^2+r2_M(2)^2];
I_M3 = m_M*[ r3_M(2)^2+r3_M(3)^2,r3_M(1)*r3_M(2),r3_M(1)*r3_M(3);...
            r3_M(1)*r3_M(2), r3_M(1)^2+r3_M(3)^2, r3_M(2)*r3_M(3);...
            r3_M(1)*r3_M(3),r3_M(2)*r3_M(3), r3_M(1)^2+r3_M(2)^2];

I_M = I_M1+I_M2+I_M3;

== matlab function NDI_and_CA_Model/3Copter_4_NDI&CA/Perturbations ==
  data: Ctrl_input_rad output; epsilon input; Ctrl_input_deg input; Pert_Ctrl_rad output
function [Ctrl_input_rad,Pert_Ctrl_rad] = Perturbate_input(epsilon, Ctrl_input_deg)
% The control input has a dimension of 9
% The gradient is computed with 2 evaluations, so the output vector has
% 2*9*9 variables

Ctrl_input_rad = Ctrl_input_deg;
Ctrl_input_rad(2:3,1) = deg2rad( Ctrl_input_deg(2:3,1) );
Ctrl_input_rad(5:6,1) = deg2rad( Ctrl_input_deg(5:6,1) );
Ctrl_input_rad(8:9,1) = deg2rad( Ctrl_input_deg(8:9,1) );

Pert_Ctrl_rad=zeros(2*9*9,1);

for i=1:9
    % Left
    tmp=Ctrl_input_rad;
    tmp(i)=tmp(i)-epsilon;
    Pert_Ctrl_rad( 1+2*(i-1)*9:(2*i-1)*9 ) = tmp;
    % Right
    tmp=Ctrl_input_rad;
    tmp(i)=tmp(i)+epsilon;
    Pert_Ctrl_rad( 1+(2*i-1)*9 :2*i*9 ) = tmp;
end






end

== matlab function NDI_and_CA_Model/3Copter_SIMPL&GRAD/Aerodynamics body Force and Moment1 ==
  data: V_b input; F_a_b output; M_a_b output; rho parameter; C_x parameter; C_y parameter; C_z parameter; A_x parameter; A_y parameter; A_z parameter
function [F_a_b,M_a_b]   = Aero_body_Forces_and_Mom( V_b, rho,C_x,C_y,C_z,A_x,A_y,A_z)


F_a_b=1/2.0*rho*(V_b*V_b')*[C_x*A_x;C_y*A_y;C_z*A_z].*( - V_b./(norm(V_b)+eps) );
M_a_b=[0;0;0];
end

== matlab function NDI_and_CA_Model/3Copter_SIMPL&GRAD/Mass Properties/Arm Inertia ==
  data: T1_FAFb input; T2_FAFb input; T3_FAFb input; I_M output; l parameter; h_M parameter; m_M parameter; r1_M output; r2_M output; r3_M output
function [I_M,r1_M,r2_M,r3_M]  = Arm1_inertia(T1_FAFb,T2_FAFb,T3_FAFb, l, h_M, m_M)


r1_M=[l;0;0]+T1_FAFb*[0;0;-h_M];
r2_M=[-1/2*l;sqrt(3)/2*l;0]+T2_FAFb*[0;0;-h_M];
r3_M=[-1/2*l;-sqrt(3)/2*l;0]+T3_FAFb*[0;0;-h_M];


I_M1 = m_M*[ r1_M(2)^2+r1_M(3)^2,r1_M(1)*r1_M(2),r1_M(1)*r1_M(3);...
            r1_M(1)*r1_M(2), r1_M(1)^2+r1_M(3)^2, r1_M(2)*r1_M(3);...
            r1_M(1)*r1_M(3),r1_M(2)*r1_M(3), r1_M(1)^2+r1_M(2)^2];
I_M2 = m_M*[ r2_M(2)^2+r2_M(3)^2,r2_M(1)*r2_M(2),r2_M(1)*r2_M(3);...
            r2_M(1)*r2_M(2), r2_M(1)^2+r2_M(3)^2, r2_M(2)*r2_M(3);...
            r2_M(1)*r2_M(3),r2_M(2)*r2_M(3), r2_M(1)^2+r2_M(2)^2];
I_M3 = m_M*[ r3_M(2)^2+r3_M(3)^2,r3_M(1)*r3_M(2),r3_M(1)*r3_M(3);...
            r3_M(1)*r3_M(2), r3_M(1)^2+r3_M(3)^2, r3_M(2)*r3_M(3);...
            r3_M(1)*r3_M(3),r3_M(2)*r3_M(3), r3_M(1)^2+r3_M(2)^2];

I_M = I_M1+I_M2+I_M3;

== matlab function NDI_and_CA_Model/3Copter_4_SIMPL/6dof Eqs of motion/SV_F_b_to_SV_FI ==
  data: q input; V_b input; V_e output
function V_e= SV_F_b_to_SV_FI(  q,V_b)

xp=V_b(1);
yp=V_b(2);
zp=V_b(3);

%% Velocity and position in Earth Frame   q . v . q*

SolProd=HamiltonProduct([q(1);q(2);q(3);q(4)],HamiltonProduct([0;xp;yp;zp],[q(1);-q(2);-q(3);-q(4)]) );
V_e=SolProd(2:4);


end

== matlab function NDI_and_CA_Model/3Copter_4_SIMPL/Mass Properties/Arm Inertia ==
  data: T1_FAFb input; T2_FAFb input; T3_FAFb input; I_M output; l parameter; h_M parameter; m_M parameter; r1_M output; r2_M output; r3_M output
function [I_M,r1_M,r2_M,r3_M]  = Arm1_inertia(T1_FAFb,T2_FAFb,T3_FAFb, l, h_M, m_M)


r1_M=[l;0;0]+T1_FAFb*[0;0;-h_M];
r2_M=[-1/2*l;sqrt(3)/2*l;0]+T2_FAFb*[0;0;-h_M];
r3_M=[-1/2*l;-sqrt(3)/2*l;0]+T3_FAFb*[0;0;-h_M];


I_M1 = m_M*[ r1_M(2)^2+r1_M(3)^2,r1_M(1)*r1_M(2),r1_M(1)*r1_M(3);...
            r1_M(1)*r1_M(2), r1_M(1)^2+r1_M(3)^2, r1_M(2)*r1_M(3);...
            r1_M(1)*r1_M(3),r1_M(2)*r1_M(3), r1_M(1)^2+r1_M(2)^2];
I_M2 = m_M*[ r2_M(2)^2+r2_M(3)^2,r2_M(1)*r2_M(2),r2_M(1)*r2_M(3);...
            r2_M(1)*r2_M(2), r2_M(1)^2+r2_M(3)^2, r2_M(2)*r2_M(3);...
            r2_M(1)*r2_M(3),r2_M(2)*r2_M(3), r2_M(1)^2+r2_M(2)^2];
I_M3 = m_M*[ r3_M(2)^2+r3_M(3)^2,r3_M(1)*r3_M(2),r3_M(1)*r3_M(3);...
            r3_M(1)*r3_M(2), r3_M(1)^2+r3_M(3)^2, r3_M(2)*r3_M(3);...
            r3_M(1)*r3_M(3),r3_M(2)*r3_M(3), r3_M(1)^2+r3_M(2)^2];

I_M = I_M1+I_M2+I_M3;
